simulink model "Motor_Model"  (Simulink 7.9)
settings: Solver=ode45  StartTime=0.0  StopTime=150  RelTol=1e-3
InitFcn:
  | Ts=0.05
libraries: simulink x1
settings Model: Creator=maen  LastModifiedBy=MAR
settings DebuggingCC: FcnCallInpInsideContextMsg=Use local settings
settings GRTTargetCC: CombineOutputUpdateFcns=off  GRTInterface=on

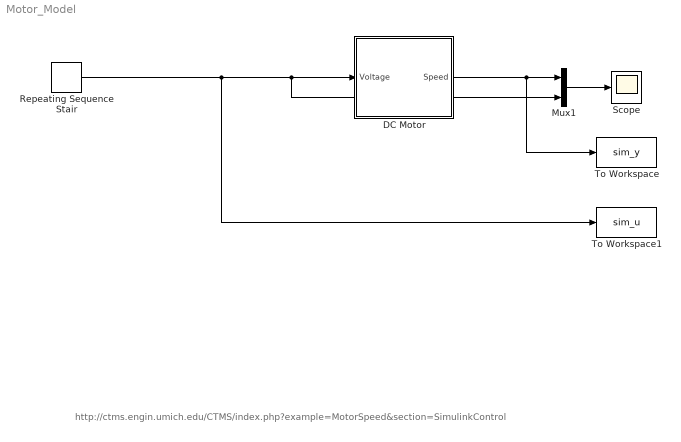
== system Motor_Model ==
  note: http://ctms.engin.umich.edu/CTMS/index.php?example=MotorSpeed&section=SimulinkControl
  DC Motor : Subsystem  mask{J=0.04, b=0.2, K=0.2775, L=0.8, R=1}
      mask prompts: J "Inertia"; b "Damping constant"; L "Inductance"; R "Resistance"
  Mux1 : Mux  Inputs=2
  Repeating Sequence Stair : simulink/Sources/Repeating Sequence Stair  OutValues=[-1 0 10 20 5 2 4 0 3 1 5 1.5 4.5 0.5 3.5 5 2.5].'  tsamp=5  OutMin=[]  OutMax=[]  OutDataTypeStr=double  OutputDataTypeScalingMode=double  OutDataType=fixdt(0,8)  ConRadixGroup=Best Precision: Vector-wise  OutScaling=2^-12
  Scope : Scope
  To Workspace : ToWorkspace  VariableName=sim_y  SampleTime=Ts
  To Workspace1 : ToWorkspace  VariableName=sim_u  SampleTime=Ts
  wires:
  Repeating Sequence Stair/1 -> To Workspace1/1, DC Motor/1(Voltage), Mux1/2
  DC Motor/1(" Speed") -> To Workspace/1, Mux1/1
  Mux1/1 -> Scope/1

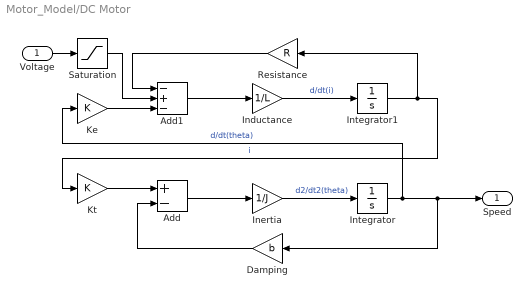
== system Motor_Model/DC Motor ==
  Voltage : Inport
  Add : Sum  Inputs=+-
  Add1 : Sum  Inputs=-+-
  Damping : Gain  Gain=b
  Inductance : Gain  Gain=1/L
  Inertia : Gain  Gain=1/J
  Integrator : Integrator
  Integrator1 : Integrator
  Ke : Gain  Gain=K
  Kt : Gain  Gain=K
  Resistance : Gain  Gain=R
  Saturation : Saturate  UpperLimit=5  LowerLimit=0
  " Speed" : Outport
  wires:
  Integrator1/1 -> Kt/1, Resistance/1  "i"
  Inductance/1 -> Integrator1/1  "d/dt(i)"
  Inertia/1 -> Integrator/1  "d2/dt2(theta)"
  Integrator/1 -> Ke/1, Damping/1, " Speed"/1  "d/dt(theta)"
  Add1/1 -> Inductance/1
  Add/1 -> Inertia/1
  Damping/1 -> Add/2
  Kt/1 -> Add/1
  Resistance/1 -> Add1/1
  Ke/1 -> Add1/3
  Voltage/1 -> Saturation/1
  Saturation/1 -> Add1/2
